simulink model "dB_lookup_table"  (R2020b)
settings: Solver=FixedStepAuto  StartTime=0.0  StopTime=stop_time  RelTol=1e-3
values from neighbouring files (symbols this model uses):
  binaryOffset = ceil(log2(maxInput))    [dB_lookup_table_sim_init.m]
  F_bits = 32    [dB_lookup_table_sim_init.m]
  M_bits = M_bits+1    (= 7)    [dB_lookup_table_sim_init.m]
  minVal = 2^(binaryOffset-(2^N_bits-1))    [dB_lookup_table_sim_init.m]
  N_bits = ceil(log2(binaryOffset-log2(floorParam)+1))    [dB_lookup_table_sim_init.m]
  ram_size = 8    [dB_lookup_table_sim_init.m]
  Table_Init = tableInit    [dB_lookup_table_sim_init.m]
libraries: FPGA_Open_Speech_Tools x3, hdlsllib x3, simulink x2
settings Model: Creator=t96f346  LastModifiedBy=conno
settings DataIOCC: SaveOutput=off  SaveTime=off  ReturnWorkspaceOutputs=off
settings OptimizationCC: DefaultParameterBehavior=Inlined

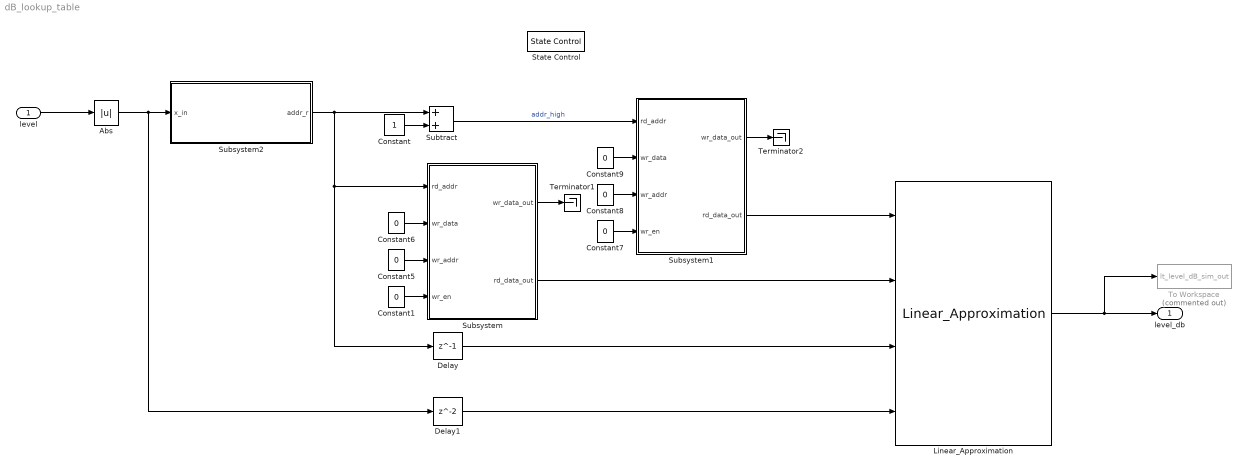
== system dB_lookup_table ==
  level : Inport  OutDataTypeStr=input_type  PortDimensions=1
  Abs : Abs
  Constant : Constant  OutDataTypeStr=fixdt(0,RAM_SIZE,0)  SampleTime=-1
  Constant1 : Constant  Value=0  OutDataTypeStr=boolean  SampleTime=-1
  Constant5 : Constant  Value=0  OutDataTypeStr=uint16  SampleTime=-1
  Constant6 : Constant  Value=0  OutDataTypeStr=input_type  SampleTime=-1
  Constant7 : Constant  Value=0  OutDataTypeStr=boolean  SampleTime=-1
  Constant8 : Constant  Value=0  OutDataTypeStr=uint16  SampleTime=-1
  Constant9 : Constant  Value=0  OutDataTypeStr=input_type  SampleTime=-1
  Delay : Delay  DelayLength=1  InitialCondition=144
  Delay1 : Delay  InitialCondition=0.0001265
  Linear_Approximation : FPGA_Open_Speech_Tools/Programmable Lookup Table dB/Linear_Approximation  SystemSampleTime=-1  VariantActivationTime=update diagram  Latency=0  AutoFrameSizeCalculation=off
  State Control : StateControl  StateControl=Synchronous
  Subsystem : Subsystem
  Subsystem1 : Subsystem
  Subsystem2 : Subsystem
  Subtract : Sum  OutDataTypeStr=Inherit: Same as first input
  Terminator1 : Terminator
  Terminator2 : Terminator
  To Workspace : ToWorkspace  Commented=on  VariableName=lt_level_dB_sim_out  SampleTime=-1
  level_db : Outport  PortDimensions=1
  wires:
  Abs/1 -> Delay1/1, Subsystem2/1(x_in)
  Constant/1 -> Subtract/2
  Delay/1 -> Linear_Approximation/3
  level/1 -> Abs/1
  Linear_Approximation/1 -> To Workspace/1, level_db/1
  Delay1/1 -> Linear_Approximation/4
  Subsystem2/1(addr_r) -> Subsystem/1(rd_addr), Delay/1, Subtract/1
  Constant6/1 -> Subsystem/2(wr_data)
  Constant5/1 -> Subsystem/3(wr_addr)
  Constant1/1 -> Subsystem/4(wr_en)
  Subsystem/1(wr_data_out) -> Terminator1/1
  Constant7/1 -> Subsystem1/4(wr_en)
  Constant8/1 -> Subsystem1/3(wr_addr)
  Constant9/1 -> Subsystem1/2(wr_data)
  Subsystem1/1(wr_data_out) -> Terminator2/1
  Subtract/1 -> Subsystem1/1(rd_addr)  "addr_high"
  Subsystem/2(rd_data_out) -> Linear_Approximation/2
  Subsystem1/2(rd_data_out) -> Linear_Approximation/1

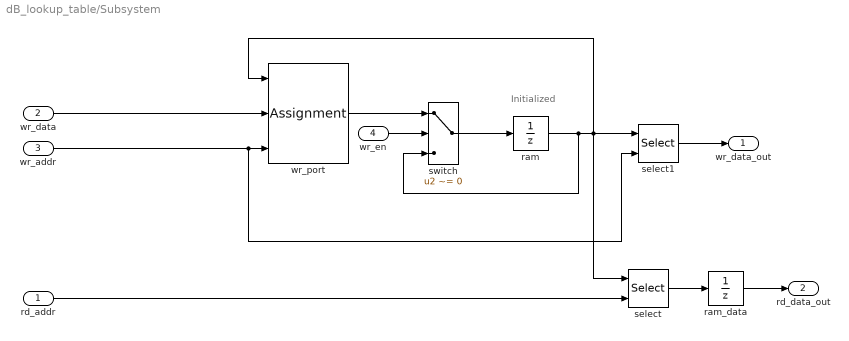
== system dB_lookup_table/Subsystem ==
  note: Initialized
  rd_addr : Inport
  wr_data : Inport  Port=2
  wr_addr : Inport  Port=3
  wr_en : Inport  Port=4  OutDataTypeStr=boolean
  ram : UnitDelay  InitialCondition=Table_Init  SampleTime=-1  HasFrameUpgradeWarning=on
  ram_data : UnitDelay  InitialCondition=55.36  SampleTime=-1  HasFrameUpgradeWarning=on
  select : Selector  IndexMode=Zero-based  InputPortWidth=2^ram_size  IndexOptions=Index vector (port)  Indices=[1 3]  OutputSizes=1
  select1 : Selector  IndexMode=Zero-based  InputPortWidth=2^ram_size  IndexOptions=Index vector (port)  Indices=[1 3]  OutputSizes=1
  switch : Switch  Criteria=u2 ~= 0
  wr_port : Assignment  IndexMode=Zero-based  IndexOptions=Index vector (port)  Indices=1  OutputSizes=[1 1]
  wr_data_out : Outport  VectorParamsAs1DForOutWhenUnconnected=off
  rd_data_out : Outport  Port=2  VectorParamsAs1DForOutWhenUnconnected=off
  wires:
  ram_data/1 -> rd_data_out/1
  wr_port/1 -> switch/1
  rd_addr/1 -> select/2
  wr_en/1 -> switch/2
  select/1 -> ram_data/1
  wr_data/1 -> wr_port/2
  ram/1 -> switch/3, select1/1, select/1, wr_port/1
  wr_addr/1 -> select1/2, wr_port/3
  switch/1 -> ram/1
  select1/1 -> wr_data_out/1

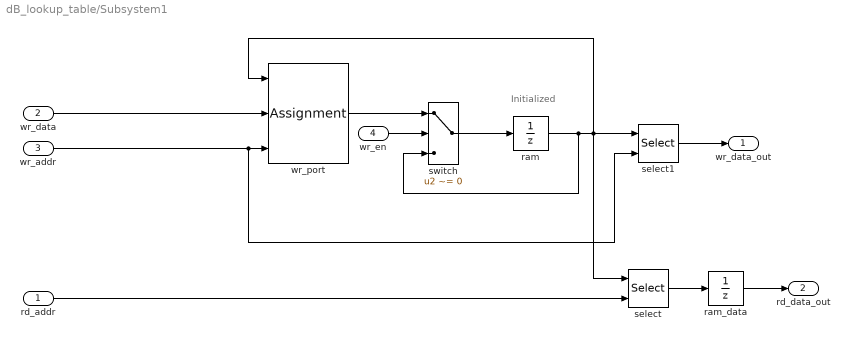
== system dB_lookup_table/Subsystem1 ==
  note: Initialized
  rd_addr : Inport
  wr_data : Inport  Port=2
  wr_addr : Inport  Port=3
  wr_en : Inport  Port=4  OutDataTypeStr=boolean
  ram : UnitDelay  InitialCondition=Table_Init  SampleTime=-1  HasFrameUpgradeWarning=on
  ram_data : UnitDelay  InitialCondition=55.36  SampleTime=-1  HasFrameUpgradeWarning=on
  select : Selector  IndexMode=Zero-based  InputPortWidth=2^ram_size  IndexOptions=Index vector (port)  Indices=[1 3]  OutputSizes=1
  select1 : Selector  IndexMode=Zero-based  InputPortWidth=2^ram_size  IndexOptions=Index vector (port)  Indices=[1 3]  OutputSizes=1
  switch : Switch  Criteria=u2 ~= 0
  wr_port : Assignment  IndexMode=Zero-based  IndexOptions=Index vector (port)  Indices=1  OutputSizes=[1 1]
  wr_data_out : Outport  VectorParamsAs1DForOutWhenUnconnected=off
  rd_data_out : Outport  Port=2  VectorParamsAs1DForOutWhenUnconnected=off
  wires:
  ram_data/1 -> rd_data_out/1
  wr_port/1 -> switch/1
  rd_addr/1 -> select/2
  wr_en/1 -> switch/2
  select/1 -> ram_data/1
  wr_data/1 -> wr_port/2
  ram/1 -> switch/3, select1/1, select/1, wr_port/1
  wr_addr/1 -> select1/2, wr_port/3
  switch/1 -> ram/1
  select1/1 -> wr_data_out/1

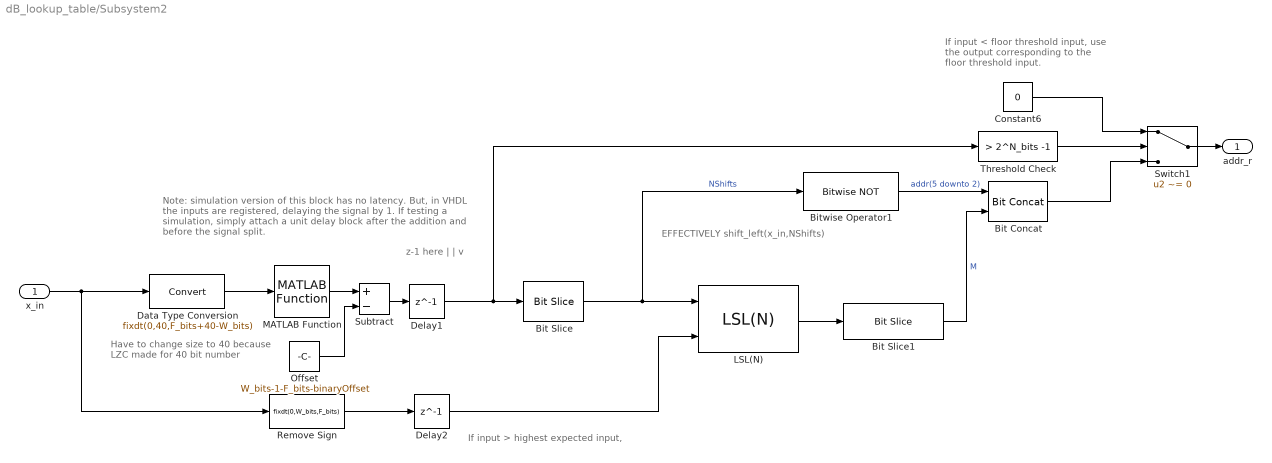
== system dB_lookup_table/Subsystem2 ==
  note: If input > highest expected input,
  note: Note: simulation version of this block has no latency.
      | But, in VHDL the inputs are registered, delaying the signal by 1.
      | If testing a simulation, simply attach a unit delay block after the
      | addition and before the signal split.
  note: If input < floor threshold input,
      | use the output corresponding to
      | the floor threshold input.
  note: z-1 here
      |    	|
      |    	|
      |   	v
  note: EFFECTIVELY shift_left(x_in,NShifts)
  note: Have to change size to 40 because
      |  LZC made for 40 bit number
  x_in : Inport
  Bit Concat : hdlsllib/Logic and Bit Operations/Bit Concat  numInputs=2
  Bit Slice : hdlsllib/Logic and Bit Operations/Bit Slice  lidx=N_bits-1  ridx=0
      settings: SourceProductBaseCode=SL
  Bit Slice1 : hdlsllib/Logic and Bit Operations/Bit Slice  lidx=F_bits-1+binaryOffset  ridx=F_bits-M_bits+binaryOffset
      settings: SourceProductBaseCode=SL
  Bitwise Operator1 : simulink/Logic and Bit Operations/Bitwise Operator  logicop=NOT  UseBitMask=off  BitMask=bin2dec('11011001')  BitMaskRealWorld=Stored Integer
  Constant6 : Constant  Value=0  OutDataTypeStr=fixdt(0,RAM_SIZE,0)  SampleTime=-1
  Data Type Conversion : DataTypeConversion  OutDataTypeStr=fixdt(0,40,F_bits+40-W_bits)
  Delay1 : Delay  DelayLength=1  InitialCondition=minVal
  Delay2 : Delay  DelayLength=1  InitialCondition=minVal
  LSL(N) : FPGA_Open_Speech_Tools/Programmable Lookup Table dB/LogAddressing/LSL(N)  SystemSampleTime=-1  VariantActivationTime=update diagram  Latency=0  AutoFrameSizeCalculation=off
  MATLAB Function : FPGA_Open_Speech_Tools/Programmable Lookup Table dB/LogAddressing/MATLAB Function  SystemSampleTime=-1  VariantActivationTime=update diagram  Latency=0  AutoFrameSizeCalculation=off
  Offset : Constant  Value=W_bits-1-F_bits-binaryOffset  OutDataTypeStr=fixdt(0,6,0)  SampleTime=-1
  Remove Sign : DataTypeConversion  OutDataTypeStr=fixdt(0,W_bits,F_bits)
  Subtract : Sum  Inputs=+-  OutDataTypeStr=Inherit: Same as first input
  Switch1 : Switch  Criteria=u2 ~= 0  OutDataTypeStr=uint8
  Threshold Check : simulink/Logic and Bit Operations/Compare To Constant  relop=>  const=2^N_bits -1  OutDataTypeStr=boolean
  addr_r : Outport  VectorParamsAs1DForOutWhenUnconnected=off
  wires:
  Offset/1 -> Subtract/2
  Bit Slice1/1 -> Bit Concat/2  "M"
  x_in/1 -> Data Type Conversion/1, Remove Sign/1
  Bit Concat/1 -> Switch1/3
  Switch1/1 -> addr_r/1
  Delay2/1 -> LSL(N)/2
  Subtract/1 -> Delay1/1
  Remove Sign/1 -> Delay2/1
  Constant6/1 -> Switch1/1
  Data Type Conversion/1 -> MATLAB Function/1
  Bit Slice/1 -> LSL(N)/1, Bitwise Operator1/1  "NShifts"
  LSL(N)/1 -> Bit Slice1/1
  Bitwise Operator1/1 -> Bit Concat/1  "addr(5 downto 2)"
  MATLAB Function/1 -> Subtract/1
  Delay1/1 -> Bit Slice/1, Threshold Check/1
  Threshold Check/1 -> Switch1/2
